simulink subsystem "OS_model"  (R2023b)
settings: Solver=VariableStepAuto  StartTime=0.0  StopTime=10.0  RelTol=1e-3
values from neighbouring files (symbols this model uses):
  l = 44.9251246151    [mdl_parameters_int.mat]
  tau_s = 0.0005    [mdl_parameters_int.mat]
settings Model: Creator=Previ  LastModifiedBy=Previ

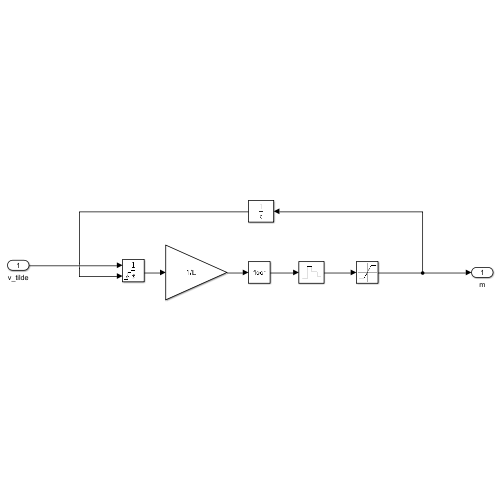
[thumbnail: Simulink's stored preview of the top-level diagram]
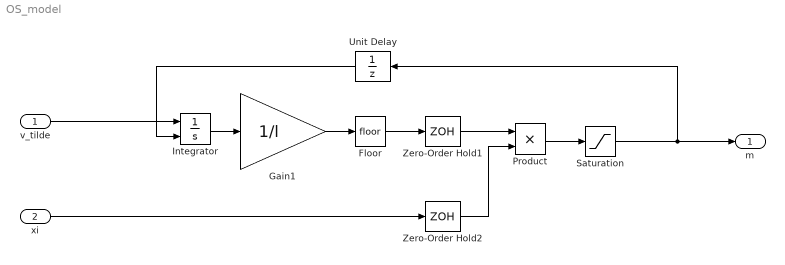
== system OS_model ==
  v_tilde : Inport  PortDimensions=[1, 1]
  xi : Inport  Port=2  PortDimensions=[1, 1]
  Floor : Rounding
  Gain1 : Gain  Gain=1/l
  Integrator : Integrator  ExternalReset=rising
  Product : Product
  Saturation : Saturate  UpperLimit=1  LowerLimit=0
  Unit Delay : UnitDelay  SampleTime=tau_s  HasFrameUpgradeWarning=on
  Zero-Order Hold1 : ZeroOrderHold  SampleTime=tau_s
  Zero-Order Hold2 : ZeroOrderHold  SampleTime=tau_s
  m : Outport  PortDimensions=[1, 1]
  wires:
  Saturation/1 -> m/1, Unit Delay/1
  Unit Delay/1 -> Integrator/2
  Floor/1 -> Zero-Order Hold1/1
  Gain1/1 -> Floor/1
  Integrator/1 -> Gain1/1
  Zero-Order Hold1/1 -> Product/1
  v_tilde/1 -> Integrator/1
  xi/1 -> Zero-Order Hold2/1
  Product/1 -> Saturation/1
  Zero-Order Hold2/1 -> Product/2
